simulink model "ff3_ff7_X3_4_7_8"  (R2015b)
settings: Solver=VariableStepAuto  StartTime=0.0  StopTime=10.0  RelTol=1e-3
undefined symbols (not defined in the file): a, alpha, beta, c, d, gama, Ps, S, tao, Ufl, Ufr
settings Model: Creator=Guest  LastModifiedBy=Guest

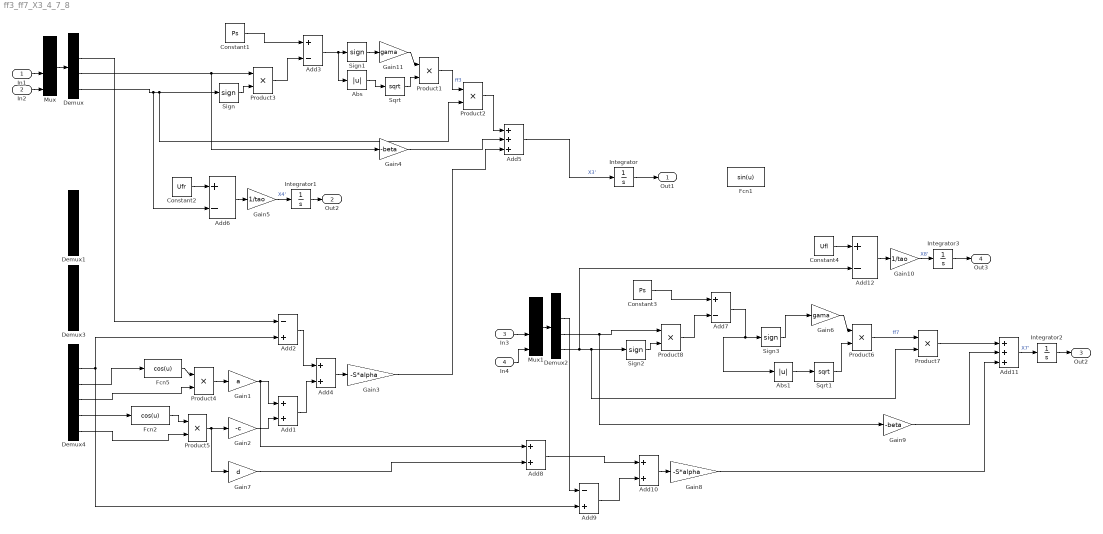
== system ff3_ff7_X3_4_7_8 ==
  In1 : Inport
  In2 : Inport  Port=2
  In3 : Inport  Port=3
  In4 : Inport  Port=4
  Abs : Abs
  Abs1 : Abs
  Add{1,4,8,10} (4 alike) : Sum
  Add11 : Sum  Inputs=+++
  Add{3,6..7,12} (4 alike) : Sum  Inputs=+-
  Add2 : Sum  Inputs=-+
  Add5 : Sum  Inputs=+++
  Add9 : Sum  Inputs=-+
  Constant1 : Constant  Value=Ps
  Constant2 : Constant  Value=Ufr
  Constant3 : Constant  Value=Ps
  Constant4 : Constant  Value=Ufl
  Demux{,1..3} (4 alike) : Demux
  Demux4 : Demux  Outputs=6
  Fcn1 : Fcn  Expr=sin(u)
  Fcn2 : Fcn  Expr=cos(u)
  Fcn5 : Fcn  Expr=cos(u)
  Gain1 : Gain  Gain=a
  Gain10 : Gain  Gain=1/tao
  Gain11 : Gain  Gain=gama
  Gain2 : Gain  Gain=-c
  Gain3 : Gain  Gain=-S*alpha
  Gain4 : Gain  Gain=-beta
  Gain5 : Gain  Gain=1/tao
  Gain6 : Gain  Gain=gama
  Gain7 : Gain  Gain=d
  Gain8 : Gain  Gain=-S*alpha
  Gain9 : Gain  Gain=-beta
  Integrator{,1..3} (4 alike) : Integrator
  Mux : Mux
  Mux1 : Mux
  Product{1..8} (8 alike) : Product
  Sign{,1..3} (4 alike) : Signum
  Sqrt : Sqrt  SaturateOnIntegerOverflow=on
  Sqrt1 : Sqrt  SaturateOnIntegerOverflow=on
  Out1 : Outport
  "Out2 " : Outport  Port=2
  Out2 : Outport  Port=3
  Out3 : Outport  Port=4
  wires:
  Demux/4 -> Add6/2, Product2/2, Sign/1
  Constant1/1 -> Add3/1
  Product3/1 -> Add3/2
  Add3/1 -> Abs/1, Sign1/1
  Sign1/1 -> Gain11/1
  Abs/1 -> Sqrt/1
  Gain11/1 -> Product1/1
  Sqrt/1 -> Product1/2
  Demux/3 -> Gain4/1, Product3/1
  Sign/1 -> Product3/2
  Product1/1 -> Product2/1  "ff3"
  Demux4/3 -> Fcn5/1
  Fcn5/1 -> Product4/1
  Demux4/4 -> Product4/2
  Product4/1 -> Gain1/1
  Demux4/5 -> Fcn2/1
  Fcn2/1 -> Product5/1
  Demux4/6 -> Product5/2
  Product5/1 -> Gain7/1, Gain2/1
  Gain2/1 -> Add1/2
  Gain1/1 -> Add8/1, Add1/1
  Demux4/2 -> Add2/2, Add9/2
  Demux/2 -> Add2/1
  Add2/1 -> Add4/1
  Add1/1 -> Add4/2
  Add4/1 -> Gain3/1
  Product2/1 -> Add5/1
  Gain4/1 -> Add5/2
  Gain3/1 -> Add5/3
  Add5/1 -> Integrator/1  "X3'"
  Integrator/1 -> Out1/1
  Mux/1 -> Demux/1
  In1/1 -> Mux/3
  Constant2/1 -> Add6/1
  Add6/1 -> Gain5/1
  Gain5/1 -> Integrator1/1  "X4'"
  Integrator1/1 -> "Out2 "/1
  In2/1 -> Mux/4
  Demux2/4 -> Add12/2, Product7/2, Sign2/1
  Constant3/1 -> Add7/1
  Product8/1 -> Add7/2
  Add7/1 -> Abs1/1, Sign3/1
  Sign3/1 -> Gain6/1
  Gain6/1 -> Product6/1
  Sqrt1/1 -> Product6/2
  Sign2/1 -> Product8/2
  Product6/1 -> Product7/1  "ff7"
  Demux2/3 -> Gain9/1, Product8/1
  Abs1/1 -> Sqrt1/1
  Gain7/1 -> Add8/2
  Demux2/2 -> Add9/1
  Add9/1 -> Add10/2
  Add8/1 -> Add10/1
  Add10/1 -> Gain8/1
  Product7/1 -> Add11/1
  Gain9/1 -> Add11/2
  Gain8/1 -> Add11/3
  Add11/1 -> Integrator2/1  "X7'"
  Integrator2/1 -> Out2/1
  Mux1/1 -> Demux2/1
  In3/1 -> Mux1/3
  Constant4/1 -> Add12/1
  Add12/1 -> Gain10/1
  Gain10/1 -> Integrator3/1  "X8'"
  Integrator3/1 -> Out3/1
  In4/1 -> Mux1/4
